simulink model "Combined"  (R2021a)
settings: Solver=VariableStepAuto  StartTime=0.0  StopTime=30.0*60*60  RelTol=1e-3
values from neighbouring files (symbols this model uses):
  A = length_of_wing^2*3.14 * number_of_windturbines    (= 78.5)    [load_global_variables.m]
  Efficiency_wind = 0.4    [load_global_variables.m]
  number_households = 200000    [load_global_variables.m]
  Rho = 1.204    [load_global_variables.m]
undefined symbols (not defined in the file or in its folder): Ion, Lithium, price, solarOneDay, time, V2G, wind
libraries: spsIdealSwitchLib x4, spsBatteryLib x1, spsDCVoltageSourceLib x1, spsSeriesRLCLoadLib x1, spspowerguiLib x1
settings Model: Creator=cm  LastModifiedBy=emilm

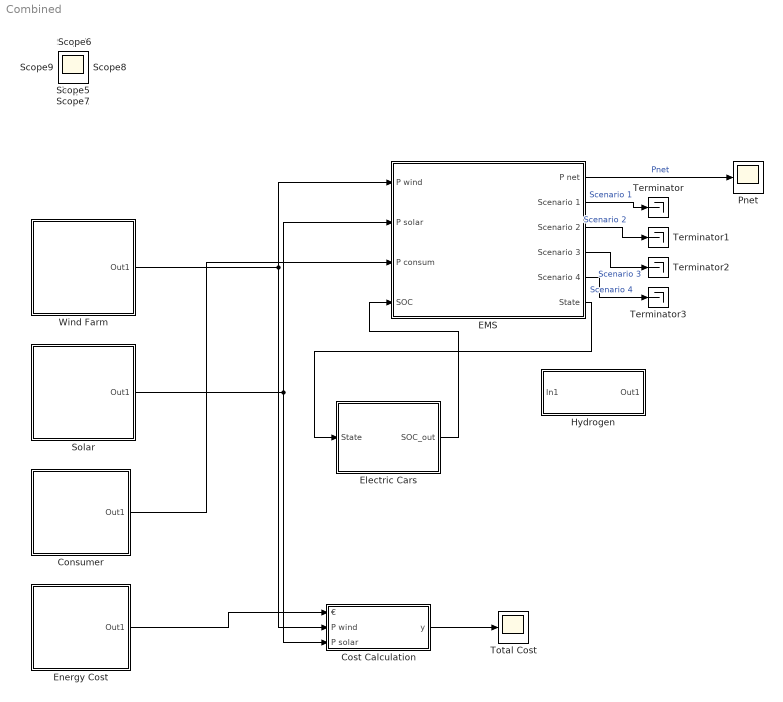
== system Combined ==
  Consumer : Subsystem
      mask Display: image('C:\Users\cm\OneDrive - Danmarks Tekniske Universitet\Model-Based Systems Eng\05 Models\OurModel\Icons\House.png'); % Use "Edit Image" on toolstrip to change.
  Cost Calculation : Subsystem
  EMS : Subsystem
  Electric Cars : Subsystem
      mask Display: image('C:\Users\cm\OneDrive - Danmarks Tekniske Universitet\Model-Based Systems Eng\05 Models\OurModel\Icons\battery.png'); % Use "Edit Image" on toolstrip to change.
  Energy Cost : Subsystem
      mask Display: image('C:\Users\cm\OneDrive - Danmarks Tekniske Universitet\Model-Based Systems Eng\05 Models\MBSE-MicroGrid\OurModel\Icons\el_cost.png'); % Use "Edit Image" on toolstrip to change.
  Hydrogen : Subsystem
  Pnet : Scope
  Solar : Subsystem
      mask Display: image('C:\Users\cm\OneDrive - Danmarks Tekniske Universitet\Model-Based Systems Eng\05 Models\OurModel\Icons\solar.png'); % Use "Edit Image" on toolstrip to change.
  Terminator{,1..3} (4 alike) : Terminator
  Total Cost : Scope
  Wind Farm : Subsystem
      mask Display: image('C:\Users\cm\OneDrive - Danmarks Tekniske Universitet\Model-Based Systems Eng\05 Models\OurModel\Icons\wind.png'); % Use "Edit Image" on toolstrip to change.
  Scope{,1..9} (10 alike) : Scope
  wires:
  Wind Farm/1(Out1) -> Cost Calculation/2(P wind), EMS/1(P wind)
  Solar/1(Out1) -> Cost Calculation/3(P solar), EMS/2(P solar)
  Consumer/1(Out1) -> EMS/3(P consum)
  EMS/1(P net) -> Pnet/1  "Pnet"
  Energy Cost/1(Out1) -> Cost Calculation/1(€)
  Cost Calculation/1(y) -> Total Cost/1
  EMS/2(Scenario 1) -> Terminator/1  "Scenario 1"
  EMS/3(Scenario 2) -> Terminator1/1  "Scenario 2"
  EMS/4(Scenario 3) -> Terminator2/1  "Scenario 3"
  EMS/5(Scenario 4) -> Terminator3/1  "Scenario 4"
  Electric Cars/1(SOC_out) -> EMS/4(SOC)
  EMS/6(State) -> Electric Cars/1(State)

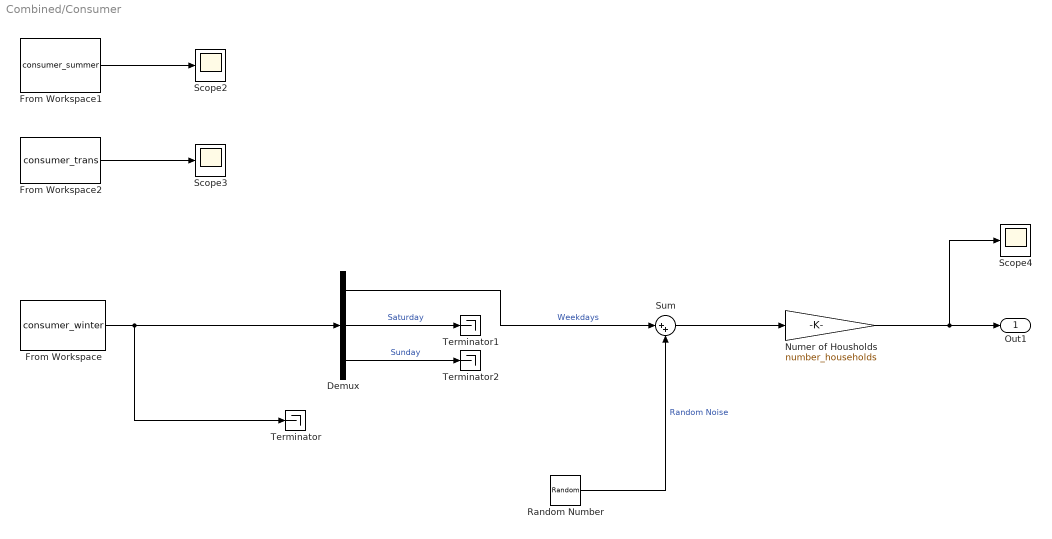
== system Combined/Consumer ==
  Demux : Demux  Outputs=3
  From Workspace : FromWorkspace  VariableName=consumer_winter  SampleTime=24*60*60/96  Interpolate=off  ZeroCross=off  OutputAfterFinalValue=Cyclic repetition
  From Workspace1 : FromWorkspace  VariableName=consumer_summer  SampleTime=24/96  Interpolate=off  ZeroCross=off  OutputAfterFinalValue=Cyclic repetition
  From Workspace2 : FromWorkspace  VariableName=consumer_trans  SampleTime=24/96  Interpolate=off  ZeroCross=off  OutputAfterFinalValue=Cyclic repetition
  Numer of Housholds : Gain  Gain=number_households
  Random Number : RandomNumber  Variance=0.0001  SampleTime=1*60*60
  Scope2 : Scope
  Scope3 : Scope
  Scope4 : Scope
  Sum : Sum  Inputs=|++
  Terminator : Terminator
  Terminator1 : Terminator
  Terminator2 : Terminator
  Out1 : Outport
  wires:
  Demux/2 -> Terminator1/1  "Saturday"
  From Workspace/1 -> Terminator/1, Demux/1
  From Workspace2/1 -> Scope3/1
  Random Number/1 -> Sum/2  "Random Noise"
  Demux/3 -> Terminator2/1  "Sunday"
  Sum/1 -> Numer of Housholds/1
  From Workspace1/1 -> Scope2/1
  Demux/1 -> Sum/1  "Weekdays"
  Numer of Housholds/1 -> Out1/1, Scope4/1

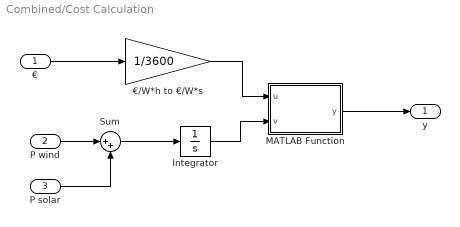
== system Combined/Cost Calculation ==
  € : Inport
  P wind : Inport  Port=2
  P solar : Inport  Port=3
  Integrator : Integrator
  MATLAB Function : MATLAB Function  TreatAsAtomicUnit=on
  Sum : Sum  Inputs=|++
  €/W*h to €/W*s : Gain  Gain=1/3600
  y : Outport
  wires:
  P wind/1 -> Sum/1
  P solar/1 -> Sum/2
  Sum/1 -> Integrator/1
  Integrator/1 -> MATLAB Function/2(v)
  MATLAB Function/1(y) -> y/1
  €/W*h to €/W*s/1 -> MATLAB Function/1(u)
  €/1 -> €/W*h to €/W*s/1

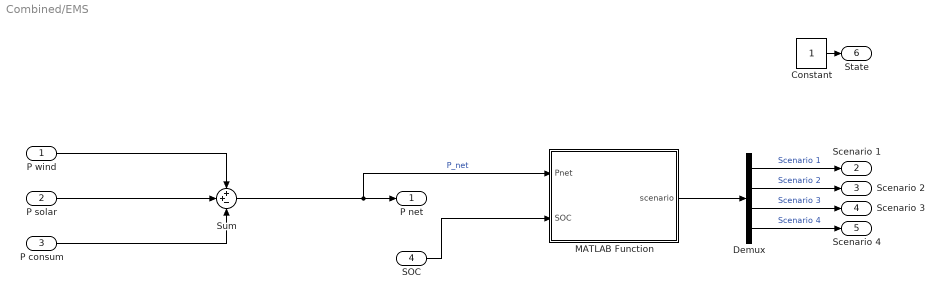
== system Combined/EMS ==
  P wind : Inport
  P solar : Inport  Port=2
  P consum : Inport  Port=3
  SOC : Inport  Port=4
  Constant : Constant
  Demux : Demux
  MATLAB Function : MATLAB Function  TreatAsAtomicUnit=on
  Sum : Sum  Inputs=++-
  P net : Outport
  Scenario 1 : Outport  Port=2
  Scenario 2 : Outport  Port=3
  Scenario 3 : Outport  Port=4
  Scenario 4 : Outport  Port=5
  State : Outport  Port=6
  wires:
  P wind/1 -> Sum/1
  P solar/1 -> Sum/2
  P consum/1 -> Sum/3
  Sum/1 -> MATLAB Function/1(Pnet), P net/1  "P_net"
  SOC/1 -> MATLAB Function/2(SOC)
  MATLAB Function/1(scenario) -> Demux/1
  Demux/1 -> Scenario 1/1  "Scenario 1"
  Demux/2 -> Scenario 2/1  "Scenario 2"
  Demux/3 -> Scenario 3/1  "Scenario 3"
  Demux/4 -> Scenario 4/1  "Scenario 4"
  Constant/1 -> State/1

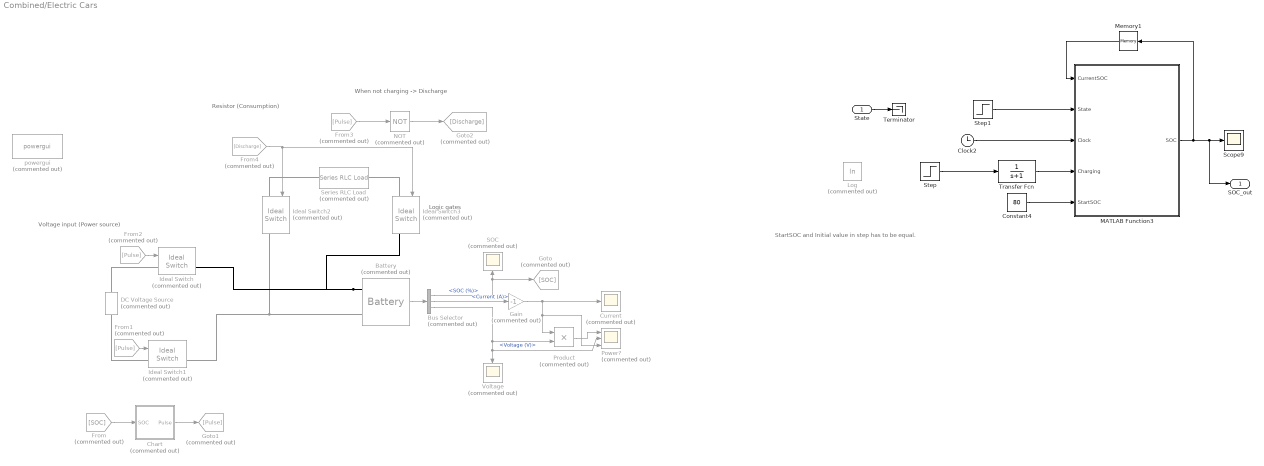
== system Combined/Electric Cars ==
  note: When not charging -> Discharge
  note: Logic gates
  note: Resistor (Consumption)
  note: Voltage input (Power source)
  note: StartSOC and Initial value in step has to be equal.
  State : Inport
  Battery : spsBatteryLib/Battery  Commented=on  BatType=Lithium-Ion  ShowTempParam=off  ThermalPreset=no  ShowAgeParam=off  NomV=7.2  NomQ=5.4  SOC=0  Batt_Tr=30  PresetModel=on  MaxQ=5.4  MinV=5.4  FullV=8.3807  Dis_rate=2.3478  R=0.013333  Normal_OP=4.8835  expZone="[7.7788      0.2653]"  current=[6.5 13 32.5]  Units=Time  Tci=20  NomT=20  T2=-30  MaxQ2=4.8  FullV2=7.1  Normal_OP2=5.655  expZone2="[6.58           1]"  Rca=0.6  ti=2000  Dp=0  Neq0=0  Tsim=1e6  Ta1=25  Qeol=5.4*0.9  Reol=0.013333*1.2  Char_age=[2.3478, 3]  Dis_age=[2.3478, 10]  N1=1500  N2=10500  N3=1000  N4=1400  Ta2=45  N5=950
  Bus Selector : BusSelector  Commented=on  OutputSignals=SOC (%),Current (A),Voltage (V)
  Chart : Stateflow chart  Commented=on  TreatAsAtomicUnit=on
  Clock2 : Clock
      settings: Decimation=100
  Constant4 : Constant  Value=80
  Current : Scope  Commented=on
  DC Voltage Source : spsDCVoltageSourceLib/DC Voltage Source  Commented=on  Amplitude=15  Measurements=None
  From : From  Commented=on  GotoTag=SOC
  From1 : From  Commented=on  GotoTag=Pulse
  From2 : From  Commented=on  GotoTag=Pulse
  From3 : From  Commented=on  GotoTag=Pulse
  From4 : From  Commented=on  GotoTag=Discharge
  Gain : Gain  Commented=on  Gain=-1
  Goto : Goto  Commented=on  GotoTag=SOC
  Goto1 : Goto  Commented=on  GotoTag=Pulse
  Goto2 : Goto  Commented=on  GotoTag=Discharge
  Ideal Switch{,1..3} (4 alike) : spsIdealSwitchLib/Ideal Switch  Commented=on  Ron=0.001  Lon=0  IC=0  Rs=1e5  Cs=inf  Measurements=on
  Log : Math  Commented=on  Operator=log  SaturateOnIntegerOverflow=on
  MATLAB Function3 : MATLAB Function  TreatAsAtomicUnit=on
  Memory1 : Memory  InheritSampleTime=on
  NOT : Logic  Commented=on  Operator=NOT  IconShape=distinctive  AllPortsSameDT=off  OutDataTypeStr=boolean
  Power? : Scope  Commented=on  NumInputPorts=3
  Product : Product  Commented=on
  SOC : Scope  Commented=on
  Scope9 : Scope
  Series RLC Load : spsSeriesRLCLoadLib/Series RLC Load  Commented=on  LConnTagsString=a  RConnTagsString=__new0  NominalVoltage=10  NominalFrequency=60  ActivePower=10e3  InductivePower=0  CapacitivePower=0  Setx0=off  InitialVoltage=0  SetiL0=off  InitialCurrent=0  Measurements=None  LoadType=constant Z
  Step : Step  Before=80  After=100  SampleTime=0
  Step1 : Step  Time=10  SampleTime=0
  Terminator : Terminator
  Transfer Fcn : TransferFcn  Denominator=[1 1]
  Voltage : Scope  Commented=on
  powergui : spspowerguiLib/powergui  Priority=1  Commented=on  SimulationMode=Continuous  SampleTime=50e-6  frequency=60  Iterations=50  frequencyindice=0  Pbase=100e6  ErrMax=1e-4  UnitsV=kV  UnitsW=MW  buscounter=0  FunctionMessages=off  echomessages=off  EnableUseOfTLC=off  CurrentSourceSwitches=off  DisableSnubberDevices=off  DisableRonSwitches=off  DisableVfSwitches=off  DisplayEquations=off  AutomaticDiscreteSolvers=off  SolverType=Tustin/Backward Euler (TBE)  Interpol=off  ExternalGateDelay=off  methode=off  Ts=100  x0status=blocks  SPID=on  SwTol=0  HookPort=off  NonlinearTolerance=1e-4  nMaxIteration=100  ContinueOnMaxIteration=off  RestoreLinks=warning  ResistiveCurrentMeasurement=off  Frange=[0:2:500]  Ylog=off  Xlog=on  ShowGrid=off  save=off  variable=ZData  structure=0  ZoomFFT=off  StartTime=0.0  cycles=1  DisplayStyle=1  fundamental=60  FreqAxis=off  MaxFrequency=1000  frequencyindicesteady=1  RmsSteady=1  display=off
  SOC_out : Outport
  wires:
  Battery/1 -> Bus Selector/1
  From2/1 -> Ideal Switch/1
  Bus Selector/2 -> Gain/1  "<Current (A)>"
  From/1 -> Chart/1(SOC)
  From1/1 -> Ideal Switch1/1
  Bus Selector/3 -> Product/2, Power?/2, Voltage/1  "<Voltage (V)>"
  From4/1 -> Ideal Switch3/1, Ideal Switch2/1
  NOT/1 -> Goto2/1
  Bus Selector/1 -> Goto/1, SOC/1  "<SOC (%)>"
  Chart/1(Pulse) -> Goto1/1
  Product/1 -> Power?/1
  From3/1 -> NOT/1
  Gain/1 -> Power?/3, Product/1, Current/1
  Constant4/1 -> MATLAB Function3/5(StartSOC)
  MATLAB Function3/1(SOC) -> SOC_out/1, Scope9/1, Memory1/1
  Clock2/1 -> MATLAB Function3/3(Clock)
  Memory1/1 -> MATLAB Function3/1(CurrentSOC)
  Step/1 -> Transfer Fcn/1
  Transfer Fcn/1 -> MATLAB Function3/4(Charging)
  State/1 -> Terminator/1
  Step1/1 -> MATLAB Function3/2(State)
  connections:
  Ideal Switch2/RConn1 -- Ideal Switch1/RConn1 -- Battery/LConn1
  Battery/LConn2 -- Ideal Switch/RConn1 -- Ideal Switch3/RConn1
  Ideal Switch3/LConn1 -- Series RLC Load/RConn1
  Ideal Switch2/LConn1 -- Series RLC Load/LConn1
  DC Voltage Source/LConn1 -- Ideal Switch/LConn1
  DC Voltage Source/RConn1 -- Ideal Switch1/LConn1

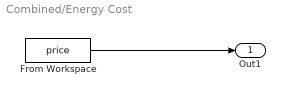
== system Combined/Energy Cost ==
  From Workspace : FromWorkspace  VariableName=price  SampleTime=24/length(price.signals.values)  Interpolate=off  ZeroCross=off  OutputAfterFinalValue=Cyclic repetition
  Out1 : Outport
  wires:
  From Workspace/1 -> Out1/1

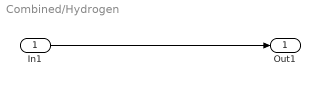
== system Combined/Hydrogen ==
  In1 : Inport
  Out1 : Outport
  wires:
  In1/1 -> Out1/1

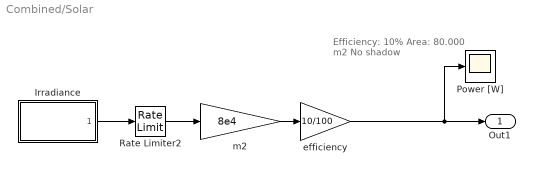
== system Combined/Solar ==
  note: Efficiency: 10%
      | Area: 80.000 m2
      | No shadow
  Irradiance : Subsystem
      mask init:
      | load power_V2G
      mask Display: plot(V2G.IRRADIANCE.time,V2G.IRRADIANCE.SUN)
  Power [W] : Scope
  Rate Limiter2 : RateLimiter  RisingSlewLimit=1e4  FallingSlewLimit=-1e4  SampleTimeMode=inherited
  efficiency : Gain  Gain=10/100
  m2 : Gain  Gain=8e4
  Out1 : Outport
  wires:
  Irradiance/1(" ") -> Rate Limiter2/1
  m2/1 -> efficiency/1
  efficiency/1 -> Out1/1, Power [W]/1
  Rate Limiter2/1 -> m2/1

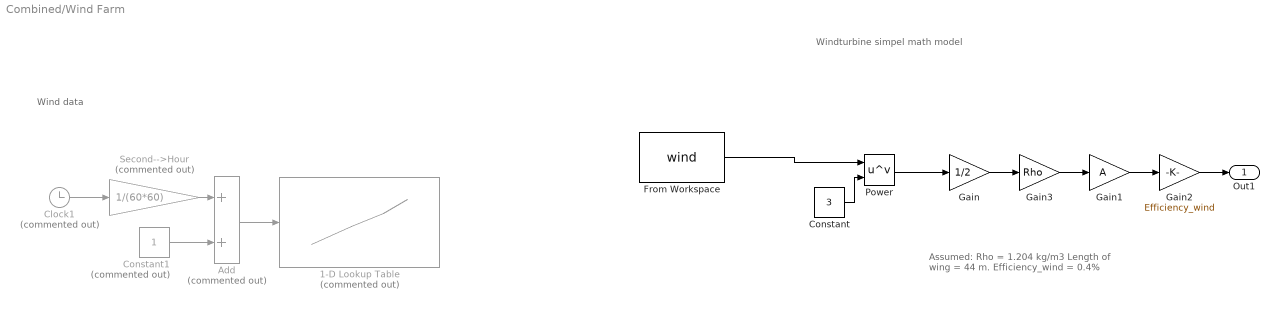
== system Combined/Wind Farm ==
  note: Assumed:
      | Rho = 1.204 kg/m3
      | Length of wing = 44 m.
      | Efficiency_wind = 0.4%
  note: Windturbine simpel math model
  note: Wind data
  1-D Lookup Table : Lookup_n-D  Commented=on  NumberOfTableDimensions=1  BreakpointsForDimension1=time  BeginIndexSearchUsingPreviousIndexResult=on  Table=wind  ExtrapMethod=Clip  UseLastTableValue=on  InternalRulePriority=Speed  RndMeth=Simplest  InputSameDT=on
  Add : Sum  Commented=on
  Clock1 : Clock  Commented=on
  Constant : Constant  Value=3
  Constant1 : Constant  Commented=on
  From Workspace : FromWorkspace  VariableName=wind  SampleTime=24*60*60/(length(wind.signals.values))  Interpolate=off  ZeroCross=off  OutputAfterFinalValue=Cyclic repetition
  Gain : Gain  Gain=1/2
  Gain1 : Gain  Gain=A
  Gain2 : Gain  Gain=Efficiency_wind
  Gain3 : Gain  Gain=Rho
  Power : Math  Operator=pow  SaturateOnIntegerOverflow=on
  Second-->Hour : Gain  Commented=on  Gain=1/(60*60)
  Out1 : Outport
  wires:
  Power/1 -> Gain/1
  Clock1/1 -> Second-->Hour/1
  Gain1/1 -> Gain2/1
  Second-->Hour/1 -> Add/1
  Add/1 -> 1-D Lookup Table/1
  Constant/1 -> Power/2
  Constant1/1 -> Add/2
  Gain/1 -> Gain3/1
  Gain3/1 -> Gain1/1
  Gain2/1 -> Out1/1
  From Workspace/1 -> Power/1

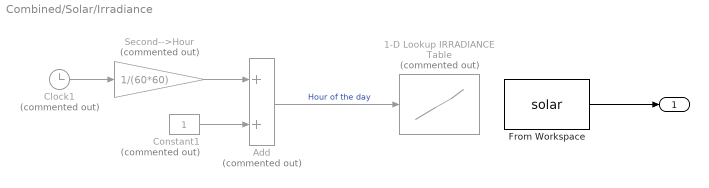
== system Combined/Solar/Irradiance ==
  1-D Lookup IRRADIANCE Table : Lookup_n-D  Commented=on  NumberOfTableDimensions=1  BreakpointsForDimension1=V2G.IRRADIANCE.time  BeginIndexSearchUsingPreviousIndexResult=on  Table=V2G.IRRADIANCE.SUN  InternalRulePriority=Speed  RndMeth=Simplest  InputSameDT=on
  Add : Sum  Commented=on
  Clock1 : Clock  Commented=on
  Constant1 : Constant  Commented=on
  From Workspace : FromWorkspace  VariableName=solar  SampleTime=24*60*60/(length(solarOneDay))  Interpolate=off  ZeroCross=off  OutputAfterFinalValue=Cyclic repetition
  Second-->Hour : Gain  Commented=on  Gain=1/(60*60)
  " " : Outport  VectorParamsAs1DForOutWhenUnconnected=off
  wires:
  Constant1/1 -> Add/2
  Add/1 -> 1-D Lookup IRRADIANCE Table/1  "Hour of the day"
  Clock1/1 -> Second-->Hour/1
  Second-->Hour/1 -> Add/1
  From Workspace/1 -> " "/1

== matlab function Combined/Cost Calculation/MATLAB Function ==
  data: u input; y output; v input
function y = multiply(u,v)

y = u*v;

== matlab function Combined/EMS/MATLAB Function ==
  data: Pnet input; scenario output; SOC input
function scenario = fcn(Pnet,SOC)

if Pnet>0
    % more engery produced than consumed
   if SOC >= 90 %TODO: global variable for SOCmax
       % Battery full
       scenario = [0 1 0 0]; %TODO: define actions for chase
   else
       % Battery not full
       scenario = [1 0 0 0]; % charge battery       
   end
else
    % more energy consumed than produced
    if SOC <= 10 %TODO: global variable for SOCmin
        % Battery empty
       scenario = [0 0 0 1]; % TODO: define actions for case. No energy in system left
    else
        % Battery not empty
        scenario = [0 0 1 0]; % discharge battery
    end
end

== stateflow chart Combined/Electric Cars/Chart ==
  state Charge
    entry : Pulse = 1
  state Discharge
    entry : Pulse = 0
  (default) -> Charge
  Charge -> Discharge : [SOC>80]
  Discharge -> Charge : [SOC<20]
  data: SOC input; Pulse output

== matlab function Combined/Electric Cars/MATLAB Function3 ==
  data: CurrentSOC input; SOC output; State input; Clock input; Charging input; StartSOC input
function SOC = fcn(CurrentSOC,State,Clock, Charging, StartSOC)




% if Clock > 30
%     
%     State = 1;
% 
% end 

% if Clock > 50
%     
%     State =2;
%     
% end

% if CurrentSOC < 50
%     
%     State = 1;
%     
% end

if State == 0 %Discharging
    if CurrentSOC == 0
        SOC = 0
    else
    
    SOC = CurrentSOC - 2;
    end
elseif State == 1 %Charging

 
     SOC = Charging;

else % Idle
    
    SOC =CurrentSOC;
    
end

if Clock == 0
    SOC = StartSOC;
end
    
end
